simulink model "mod_sim_VTMS"  (R2018b)
settings: Solver=FixedStepDiscrete  StartTime=0.0  StopTime=t_Simulation  FixedStep=delta_t  RelTol=1e-3
values from neighbouring files (symbols this model uses):
  P_charge = 150    [main_sim_VTMS.m]
undefined symbols (not defined in the file or in its folder): A_EMaschine_Getriebe, A_j_c, A_Stirn, Anzahl_Peltierelemente, b_Batteriepack, b_c, b_EMaschine, b_Getriebe, b_j, b_Ladegeraet, BatPara, c_W, delta_t, DiscIntNeverNeededParam, e_Fahrzeug, eta_EMaschine_Break_M_EMaschine, eta_EMaschine_Break_n_EMaschine, eta_EMaschine_Faktor_Volllast, eta_EMaschine_Table, eta_Getriebe, eta_Ladegeraet, eta_Leistungselektronik_Break_M_EMaschine, eta_Leistungselektronik_Break_n_EMaschine, eta_Leistungselektronik_Faktor_Volllast, eta_Leistungselektronik_Table, f_R, I_DT_U_Break_DT, I_DT_U_Break_U, I_DT_U_Value_I, i_Getriebe, I_max, Ladevorgang, M_EMaschine_max, m_Fahrzeug, m_Zuladung, n_Zelle, P_Nebenverbraucher, p_Zelle, Peltier_Max_Eff, Q_DT_U_Break_DT, Q_DT_U_Break_U, Q_DT_U_Value_Q, Q_Imax_DT_Break_DT, Q_Imax_DT_Value_Q, r_dynamisch, rho_Luft, s_Zelle, SOC_init, Steuerung_Kuehlerluefter, Steuerung_Pumpe, Steuerung_Ventil, switch_BP_Zyklus, T_Batteriepack_init, T_EMaschine_Getriebe_init, T_Ladegeraet_init, T_Ladegeraet_Offset, T_Leistungselektronik_init, T_Offset_Batteriepack, T_Offset_EMaschine_Getriebe, T_Offset_Leistungselektronik ... (+36)
libraries: simulink x3, simulink_extras x2
(part 4 of 5)

== system mod_sim_VTMS/Thermomanagementsystem/Fluid/Fluid_Komponente thermisch/Konduktion 1. finites Volumen mit vorheriger Fluid_Komponente - Ventil ==
  note: PQ_FinitesVolumen_FinitesVolumen_1 = (T_FinitesVolumen_vor1_n - T_FinitesVolumen_1) / R_Ersatz
      | = Konduktion für das 1. finite Volumen mit vorherigem finiten Volumen
      |
      | mit R_Ersatz für Hauptpfad (Hauptpfad = 1) = R_FinitesVolumen / 2 + R_FinitesVolumen_vor1 / (2 * (1 - Zustand_Ventil)) = (R_FinitesVolumen + R_FinitesVolumen_vor1 / (1 - Zustand_Ventil)) / 2
      | mit R_Ersatz für Nebenpfad (Hauptpfad = 0) = R_FinitesVolumen / 2 + R_FinitesVolumen_vor1 / (2 * Zustand_Ventil) = (R_FinitesVolumen + R_FinitesVolumen_vor1 / Zustand_Ventil) / 2
      |
      | -> Dieses Subsystem repräsentiert den Fall, dass sich diese Fluid_Komponente sich nach einem Dreiwegeventil befindet
      | -> Diese Fluid_Komponente befindet sich nach 1 Fluid_Komponente + Fluid_Komponente vor dieser Fluid_Komponente befindet sich vor 2 Fluid_Komponenten
      | -> Diese Fluid_Komponente befindet sich entweder im Hauptpfad oder im Nebenpfad dieses Dreiwegeventils
      | -> Der Anwender legt in MATLAB fest, in welchem Pfad des Dreiwegeventils sich diese Fluid_Komponente befindet
      | -> Hauptpfad: Bei Zustand_Ventil = 0 fließt alles über den Hauptpfad, bei Zustand_Ventil = 1 fließt nichts über den Hauptpfad
      | -> Nebenpfad: Bei Zustand_Ventil = 0 fließt nichts über den Nebenpfad, bei Zustand_Ventil = 1 fließt alles über den Nebenpfad
      | -> Es gilt die Annahme: Diese Fluid_Komponente steht in Beziehung mit Zustand_Ventil (falls im Nebenpfad dieses Dreiwegeventils) bzw. mit (1 - Zustand_Ventil) (falls im Hauptpfad dieses Dreiwegeventils) der Querschnittsfläche der Kühlflüssigkeit in Fluid_Komponente_vor1
      |
      | -> Für die Herleitung dieses mathematischen Zusammenhangs wird auf die auf die im Rahmen des Thermomanagementsystemmodells erstellte Masterarbeit "Entwicklung und Steuerung eines Thermomanagementsystemmodells für Elektrofahrzeuge" verwiesen
  T_FinitesVolumen [K] : Inport
  R_FinitesVolumen [K*W^-1] : Inport  Port=2
  T_FinitesVolumen_vor1 [K] : Inport  Port=3
  R_FinitesVolumen_vor1 [K*W^-1] : Inport  Port=4
  Zustand_Ventil [-] : Inport  Port=5
  Add : Sum
  Constant : Constant  VectorParams1D=off
  Divide : Product  Inputs=*/
  Gain : Gain  Gain=0.5
  Hauptpfad : Constant  Value=0  VectorParams1D=off
  MATLAB Function : MATLAB Function  TreatAsAtomicUnit=on
  Subtract : Sum  Inputs=+-
  Switch : Switch  Criteria=u2 > Threshold
  PQ_FinitesVolumen_FinitesVolumen [W] : Outport
  wires:
  MATLAB Function/1(y) -> PQ_FinitesVolumen_FinitesVolumen [W]/1
  T_FinitesVolumen_vor1 [K]/1 -> MATLAB Function/2(v)
  R_FinitesVolumen_vor1 [K*W^-1]/1 -> Divide/1
  T_FinitesVolumen [K]/1 -> MATLAB Function/1(u)
  Divide/1 -> Add/2
  R_FinitesVolumen [K*W^-1]/1 -> Add/1
  Add/1 -> Gain/1
  Gain/1 -> MATLAB Function/3(a)
  Switch/1 -> Divide/2
  Zustand_Ventil [-]/1 -> Subtract/2, Switch/3
  Subtract/1 -> Switch/1
  Constant/1 -> Subtract/1
  Hauptpfad/1 -> Switch/2

== system mod_sim_VTMS/Thermomanagementsystem/Fluid/Fluid_Komponente thermisch/Konduktion 1. finites Volumen mit vorheriger Fluid_Komponente - normal ==
  note: PQ_FinitesVolumen_FinitesVolumen_1 = (T_FinitesVolumen_vor1_n - T_FinitesVolumen_1) / R_Ersatz
      | = Konduktion für das 1. finite Volumen mit vorherigem finiten Volumen
      |
      | mit R_Ersatz = R_FinitesVolumen / 2 + R_FinitesVolumen_vor1 / 2 = (R_FinitesVolumen + R_FinitesVolumen_vor1) / 2
      |
      | -> Dieses Subsystem repräsentiert den Fall, dass sich diese Fluid_Komponente nach einer anderen Fluid_Komponente ohne Dreiwegeventil oder Vereinigung der zwei nach der Aufzweigung durch ein Dreiwegeventil resultierenden Pfade befindet
      | -> Diese Fluid_Komponente befindet sich nach 1 Fluid_Komponente + Fluid_Komponente vor dieser Fluid_Komponente befindet sich vor 1 Fluid_Komponente
      |
      | -> Für die Herleitung dieses mathematischen Zusammenhangs wird auf die auf die im Rahmen des Thermomanagementsystemmodells erstellte Masterarbeit "Entwicklung und Steuerung eines Thermomanagementsystemmodells für Elektrofahrzeuge" verwiesen
  T_FinitesVolumen [K] : Inport
  R_FinitesVolumen [K*W^-1] : Inport  Port=2
  T_FinitesVolumen_vor1 [K] : Inport  Port=3
  R_FinitesVolumen_vor1 [K*W^-1] : Inport  Port=4
  Add : Sum
  Gain : Gain  Gain=0.5
  MATLAB Function : MATLAB Function  TreatAsAtomicUnit=on
  PQ_FinitesVolumen_FinitesVolumen [W] : Outport
  wires:
  R_FinitesVolumen_vor1 [K*W^-1]/1 -> Add/2
  T_FinitesVolumen_vor1 [K]/1 -> MATLAB Function/2(v)
  MATLAB Function/1(y) -> PQ_FinitesVolumen_FinitesVolumen [W]/1
  R_FinitesVolumen [K*W^-1]/1 -> Add/1
  Add/1 -> Gain/1
  T_FinitesVolumen [K]/1 -> MATLAB Function/1(u)
  Gain/1 -> MATLAB Function/3(a)

== system mod_sim_VTMS/Thermomanagementsystem/Fluid/Fluid_Komponente thermisch/Konduktion finite Volumen innerhalb Fluid_Komponente ==
  note: PQ_FinitesVolumen_FinitesVolumen_i = (T_FinitesVolumen_i-1 - T_FinitesVolumen_i) / R_FinitesVolumen + (T_FinitesVolumen_i+1 - T_FinitesVolumen_i) / R_FinitesVolumen für i = 2 ... n-1
      | = (T_FinitesVolumen_i-1 + T_FinitesVolumen_i+1 - 2 * T_FinitesVolumen_i) / R_FinitesVolumen für i = 2 ... n-1
      | = Konduktion für das i. finite Volumen mit vorherigem und nachfolgendem finiten Volumen für i = 2 ... n-1
      |
      | PQ_FinitesVolumen_FinitesVolumen_1 = (T_FinitesVolumen_2 - T_FinitesVolumen_1) / R_FinitesVolumen
      | = Konduktion für das 1. finite Volumen mit nachfolgendem finiten Volumen
      |
      | PQ_FinitesVolumen_FinitesVolumen_n = (T_FinitesVolumen_n-1 - T_FinitesVolumen_n) / R_FinitesVolumen
      | = Konduktion für das n. finite Volumen mit vorherigem finiten Volumen
      |
      | -> Der Widerstand zwischen den einzelnen Knoten der finiten Volumen ist jeweils R_FinitesVolumen, weil die Wärmeleitfähigkeit und die Querschnittsfläche der Kühlflüssigkeit innerhalb einer Fluid_Komponente identisch sind und der Abstand zwischen den einzelnen Knoten gleich der Länge eines finiten Volumen ist
      | -> Die Bestimmung der Konduktion für ein finites Volumen mit vorherigem und nachfolgenden finiten Volumen ist innerhalb einer Fluid_Komponente nur für i = 2 ... n-1 möglich, weil das 1. bzw. n. finite Volumen einer Fluid_Komponente nur Konduktion mit dem 2. (nachfolgenden) bzw. n-1. (vorherigem) finten Volumen derselben Fluid_Komponente hat
      | -> Die restliche Konduktion für das 1. und n. finite Volumen finden mit anderen Fluid_Komponenten statt und werden deswegen durch die Kopplungsfälle dargestellt
      |
      | -> Für die Herleitung dieser mathematischen Zusammenhänge wird auf die auf die im Rahmen des Thermomanagementsystemmodells erstellte Masterarbeit "Entwicklung und Steuerung eines Thermomanagementsystemmodells für Elektrofahrzeuge" verwiesen
      |
      | -> Für die Herleitung dieses mathematischen Zusammenhangs wird auf die auf die im Rahmen des Thermomanagementsystemmodells erstellte Masterarbeit "Entwicklung und Steuerung eines Thermomanagementsystemmodells für Elektrofahrzeuge" verwiesen
      | -> Für die Herleitung dieses mathematischen Zusammenhangs wird auf die auf die im Rahmen des Thermomanagementsystemmodells erstellte Masterarbeit "Entwicklung und Steuerung eines Thermomanagementsystemmodells für Elektrofahrzeuge" verwiesen
      | -> Für die Herleitung dieses mathematischen Zusammenhangs wird auf die auf die im Rahmen des Thermomanagementsystemmodells erstellte Masterarbeit "Entwicklung und Steuerung eines Thermomanagementsystemmodells für Elektrofahrzeuge" verwiesen
  T_FinitesVolumen [K] : Inport
  R_FinitesVolumen [K*W^-1] : Inport  Port=2
  MATLAB Function : MATLAB Function  TreatAsAtomicUnit=on
  PQ_FinitesVolumen_FinitesVolumen [W] : Outport
  wires:
  T_FinitesVolumen [K]/1 -> MATLAB Function/1(u)
  R_FinitesVolumen [K*W^-1]/1 -> MATLAB Function/2(a)
  MATLAB Function/1(y) -> PQ_FinitesVolumen_FinitesVolumen [W]/1

== system mod_sim_VTMS/Thermomanagementsystem/Fluid/Fluid_Komponente thermisch/Konduktion n. finites Volumen mit nachfolgenden Fluid_Komponenten - Ventil ==
  note: PQ_FinitesVolumen_FinitesVolumen_n = (T_FinitesVolumen_nach1_1 - T_FinitesVolumen_n) / R_Ersatz_1 + (T_FinitesVolumen_nach2_1 - T_FinitesVolumen_n) / R_Ersatz_2
      | = Konduktion für das n. finite Volumen mit nachfolgendem finiten Volumen
      |
      | mit R_Ersatz_1 = R_FinitesVolumen / (2 * (1 - Zustand_Ventil)) + R_FinitesVolumen_nach1 / 2 = (R_FinitesVolumen / (1 - Zustand_Ventil) + R_FinitesVolumen_nach1) / 2 -> Fluid_Komponente_nach1 befindet sich im Hauptpfad des Dreiwegeventils
      | mit R_Ersatz_2 = R_FinitesVolumen / (2 * Zustand_Ventil) + R_FinitesVolumen_nach1 / 2 = (R_FinitesVolumen / Zustand_Ventil + R_FinitesVolumen_nach2) / 2 -> Fluid_Komponente_nach2 befindet sich im Nebenpfad des Dreiwegeventils
      |
      | -> Dieses Subsystem repräsentiert den Fall, dass sich diese Fluid_Komponente vor einem Dreiwegeventil befindet
      | -> Diese Fluid_Komponente befindet sich vor 2 Fluid_Komponenten
      | -> Eine der nachfolgenden Fluid_Komponenten befindet sich im Hauptpfad dieses Dreiwegeventils und die andere nachfolgende Fluid_Komponente im Nebenpfad dieses Dreiwegeventil
      | -> Der Anwender legt in MATLAB fest, in welchem Pfad des Dreiwegeventils sich die nachfolgenden Fluid_Komponenten befinden
      | -> Fluid_Komponente_nach1 befindet sich im Hauptpfad dieses Dreiwegeventils, Fluid_Komponente_nach2 befindet sich im Nebenpfad dieses Dreiwegeventils
      | -> Hauptpfad: Bei Zustand_Ventil = 0 fließt alles über den Hauptpfad, bei Zustand_Ventil = 1 fließt nichts über den Hauptpfad
      | -> Nebenpfad: Bei Zustand_Ventil = 0 fließt nichts über den Nebenpfad, bei Zustand_Ventil = 1 fließt alles über den Nebenpfad
      | -> Es gilt die Annahme: Diese Fluid_Komponente steht mit (1 - Zustand_Ventil) ihrer Querschnittsfläche der Kühlflüssigkeit in Beziehung mit Fluid_Komponente_nach1 und mit Zustand_Ventil ihrer Querschnittsfläche der Kühlflüssigkeit in Beziehnung mit Fluid_Komponente_nach2
      |
      | -> Für die Herleitung dieses mathematischen Zusammenhangs wird auf die auf die im Rahmen des Thermomanagementsystemmodells erstellte Masterarbeit "Entwicklung und Steuerung eines Thermomanagementsystemmodells für Elektrofahrzeuge" verwiesen
  T_FinitesVolumen [K] : Inport
  R_FinitesVolumen [K*W^-1] : Inport  Port=2
  T_FinitesVolumen_nach1 [K] : Inport  Port=3
  R_FinitesVolumen_nach1 [K*W^-1] : Inport  Port=4
  T_FinitesVolumen_nach2 [K] : Inport  Port=5
  R_FinitesVolumen_nach2 [K*W^-1] : Inport  Port=6
  Zustand_Ventil [-] : Inport  Port=7
  Add : Sum
  Add1 : Sum
  Constant : Constant
  Divide : Product  Inputs=*/
  Divide1 : Product  Inputs=*/
  Gain : Gain  Gain=0.5
  Gain1 : Gain  Gain=0.5
  MATLAB Function : MATLAB Function  TreatAsAtomicUnit=on
  Subtract : Sum  Inputs=+-
  PQ_FinitesVolumen_FinitesVolumen [W] : Outport
  wires:
  R_FinitesVolumen [K*W^-1]/1 -> Divide1/1, Divide/1
  Add/1 -> Gain/1
  Divide/1 -> Add/1
  MATLAB Function/1(y) -> PQ_FinitesVolumen_FinitesVolumen [W]/1
  T_FinitesVolumen [K]/1 -> MATLAB Function/1(u)
  T_FinitesVolumen_nach2 [K]/1 -> MATLAB Function/3(w)
  T_FinitesVolumen_nach1 [K]/1 -> MATLAB Function/2(v)
  Gain/1 -> MATLAB Function/4(a)
  Subtract/1 -> Divide/2
  Constant/1 -> Subtract/1
  R_FinitesVolumen_nach1 [K*W^-1]/1 -> Add/2
  Add1/1 -> Gain1/1
  Divide1/1 -> Add1/1
  Gain1/1 -> MATLAB Function/5(b)
  R_FinitesVolumen_nach2 [K*W^-1]/1 -> Add1/2
  Zustand_Ventil [-]/1 -> Divide1/2, Subtract/2

== system mod_sim_VTMS/Thermomanagementsystem/Fluid/Fluid_Komponente thermisch/Konduktion n. finites Volumen mit nachfolgender Fluid_Komponente - Vereinigung ==
  note: PQ_FinitesVolumen_FinitesVolumen_n = (T_FinitesVolumen_nach1_1 - T_FinitesVolumen_n) / R_Ersatz
      | = Konduktion für das n. finite Volumen mit nachfolgendem finiten Volumen
      |
      | mit R_Ersatz = R_FinitesVolumen / 2 + R_FinitesVolumen_nach1 / (2 * 0.5) = R_FinitesVolumen / 2 + R_FinitesVolumen_nach1
      |
      | -> Dieses Subsystem repäsentiert den Fall, dass sich diese Fluid_Komponente vor der Vereinigung der zwei nach der Aufzweigung durch ein Dreiwegeventil resultierenden Pfade befindet
      | -> Diese Fluid_Komponente befindet sich vor 1 Fluid_Komponente + Fluid_Komponente nach dieser Fluid_Komponente befindet sich nach 2 Fluid_Komponenten
      | -> Diese Fluid_Komponente befindet sich in einem der Pfade dieses Dreiwegeventils (es ist egal, in welchem Pfad dieses Dreiwegeventils, weil das Prinzip der Berechnung gleich ist -> siehe unten)
      | -> Nach dieser Fluid_Komponente befindet sich kein Dreiwegeventil mit einem bestimmten Zustand, sondern es gilt die Annahme: Diese Fluid_Komponente steht in Beziehung mit 50% der Querschnittsfläche der Kühlflüssigkeit in Fluid_Komponente_nach1
      |
      | -> Für die Herleitung dieses mathematischen Zusammenhangs wird auf die auf die im Rahmen des Thermomanagementsystemmodells erstellte Masterarbeit "Entwicklung und Steuerung eines Thermomanagementsystemmodells für Elektrofahrzeuge" verwiesen
  T_FinitesVolumen [K] : Inport
  R_FinitesVolumen [K*W^-1] : Inport  Port=2
  T_FinitesVolumen_nach1 [K] : Inport  Port=3
  R_FinitesVolumen_nach1 [K*W^-1] : Inport  Port=4
  Add1 : Sum
  Gain1 : Gain  Gain=0.5
  MATLAB Function : MATLAB Function  TreatAsAtomicUnit=on
  PQ_FinitesVolumen_FinitesVolumen [W] : Outport
  wires:
  T_FinitesVolumen_nach1 [K]/1 -> MATLAB Function/2(v)
  MATLAB Function/1(y) -> PQ_FinitesVolumen_FinitesVolumen [W]/1
  T_FinitesVolumen [K]/1 -> MATLAB Function/1(u)
  R_FinitesVolumen_nach1 [K*W^-1]/1 -> Add1/2
  R_FinitesVolumen [K*W^-1]/1 -> Gain1/1
  Gain1/1 -> Add1/1
  Add1/1 -> MATLAB Function/3(a)

== system mod_sim_VTMS/Thermomanagementsystem/Fluid/Fluid_Komponente thermisch/Konduktion n. finites Volumen mit nachfolgender Fluid_Komponente - normal ==
  note: PQ_FinitesVolumen_FinitesVolumen_n = (T_FinitesVolumen_nach1_1 - T_FinitesVolumen_n) / R_Ersatz
      | = Konduktion für das n. finite Volumen mit nachfolgendem finiten Volumen
      |
      | mit R_Ersatz = R_FinitesVolumen / 2 + R_FinitesVolumen_nach1 / 2 = (R_FinitesVolumen + R_FinitesVolumen_nach1) / 2
      |
      | -> Dieses Subsystem repräsentiert den Fall, dass sich diese Fluid_Komponente vor einer anderen Fluid_Komponente ohne Dreiwegeventil oder Vereinigung der zwei nach der Aufzweigung durch ein Dreiwegeventil resultierenden Pfade befindet
      | -> Diese Fluid_Komponente befindet sich vor 1 Fluid_Kompnente + Fluid_Komponente nach dieser Fluid_Komponente befindet sich nach 1 Fluid_Komponente
      |
      | -> Für die Herleitung dieses mathematischen Zusammenhangs wird auf die auf die im Rahmen des Thermomanagementsystemmodells erstellte Masterarbeit "Entwicklung und Steuerung eines Thermomanagementsystemmodells für Elektrofahrzeuge" verwiesen
  T_FinitesVolumen [K] : Inport
  R_FinitesVolumen [K*W^-1] : Inport  Port=2
  T_FinitesVolumen_nach1 [K] : Inport  Port=3
  R_FinitesVolumen_nach1 [K*W^-1] : Inport  Port=4
  Add : Sum
  Gain : Gain  Gain=0.5
  MATLAB Function : MATLAB Function  TreatAsAtomicUnit=on
  PQ_FinitesVolumen_FinitesVolumen [W] : Outport
  wires:
  MATLAB Function/1(y) -> PQ_FinitesVolumen_FinitesVolumen [W]/1
  Gain/1 -> MATLAB Function/3(a)
  T_FinitesVolumen [K]/1 -> MATLAB Function/1(u)
  R_FinitesVolumen_nach1 [K*W^-1]/1 -> Add/2
  R_FinitesVolumen [K*W^-1]/1 -> Add/1
  T_FinitesVolumen_nach1 [K]/1 -> MATLAB Function/2(v)
  Add/1 -> Gain/1

== system mod_sim_VTMS/Thermomanagementsystem/Kühler/Kuehler thermisch/Bestimmung v_Kuehlerluefter ==
  note: -> Ein Kühlerlüfter wird nicht modelliert
      | -> Es wird nur die Luftgeschwindigkeit eines Kühlerlüfters benötigt
      | -> Kühlerlüfter gesteuert (Steuerung_Kuehlerluefter = 1): v_Kuehlerluefter wird über Steuerung in Subsystem "Steuerung Kuehlerluefter" bestimmt
      | -> Kühlerlüfter ungesteuert (Steuerung_Kuehlerluefter = 0): v_Kuehlerluefter wird zeitabhängig vom Anwender vorgegeben
  note: -> Ein Kühler besitzt einen Kühlerlüfter, der den Kühler mit seiner Luftgeschwindigkeit anströmt
      | -> Ein Kühlerlüfter wird als 0D angenommen
      | -> Je nachdem wie es der Anwender wünscht, können Kühlerlüfter gesteuert oder ungesteuert sein
  T_FinitesVolumen [K] : Inport
  Constant : Constant  Value=Steuerung_Kuehlerluefter  VectorParams1D=off
  Steuerung Kuehlerluefter : Subsystem
  Switch : Switch  Criteria=u2 > Threshold
  v_Kuehlerluefter : FromWorkspace  VariableName=[0,0]  SampleTime=0
  v_Kuehlerluefter [m*s^-1] : Outport
  wires:
  Switch/1 -> v_Kuehlerluefter [m*s^-1]/1
  Constant/1 -> Switch/2
  v_Kuehlerluefter/1 -> Switch/3
  Steuerung Kuehlerluefter/1(v_Kuehlerluefter [m*s^-1]) -> Switch/1
  T_FinitesVolumen [K]/1 -> Steuerung Kuehlerluefter/1(T_FinitesVolumen [K])

== system mod_sim_VTMS/Thermomanagementsystem/Ladegeraet/Ladegeraet(1) elektrisch/Fast charging control ==
  note: Current reduction step in W
      | if max voltage is reached
  U_cell [V] : Inport
  Enable : EnablePort  StatesWhenEnabling=reset
  Add1 : Sum  Inputs=+-
  Charging Power : UnitDelay  InitialCondition=P_charge*1000  SampleTime=-1
  Constant2 : Constant  Value=100
  Constant3 : Constant  Value=0
  Saturation : Saturate  UpperLimit=inf  LowerLimit=0
  Switch1 : Switch  Threshold=4.18
  charging power [W] : Outport  OutputWhenDisabled=reset  InitialOutput=0
  wires:
  Constant2/1 -> Switch1/1
  Constant3/1 -> Switch1/3
  Add1/1 -> Saturation/1
  Switch1/1 -> Add1/2
  U_cell [V]/1 -> Switch1/2
  Charging Power/1 -> Add1/1
  Saturation/1 -> charging power [W]/1, Charging Power/1

== system mod_sim_VTMS/Thermomanagementsystem/Ladegeraet/Ladegeraet(1) thermisch/Waermeaustausch Ladegeraet - Fluid ==
  note: PQ_Ladegeraet_FinitesVolumen_i = UA_Ladegeraet_FinitesVolumen * (T_Ladegeraet - T_FinitesVolumen_i) für i = 1:n
      | PQ_Ladegeraet_Kuehlfluessigkeit = Summe (PQ_Ladegeraet_FinitesVolumen_i) für i = 1:n
      |
      | mit UA_Ladegeraet_FinitesVolumen = f (PV_Kuehlfluessigkeit)
      |
      | -> UA_Ladegeraet_FinitesVolumen und T_Ladegeraet ist für jedes finite Volumen des Fluids im Ladegeraet identisch, weil das Ladegeraet als Punktmasse betrachtet wird
      |
      | -> Deswegen ergibt sich die Wärmeleistung bzgl. dem Ladegeraet über den Wärmeaustausch mit der gesamten Kühlflüssigkeit, was der Summe aus den Wärmeaustauschen mit den finiten Volumen entspricht
  T_Ladegeraet [K] : Inport
  T_FinitesVolumen [K] : Inport  Port=2
  PV_Ladegeraet [m^3*s^-1] : Inport  Port=3
  1-D Lookup Table : Lookup_n-D  NumberOfTableDimensions=1  BreakpointsForDimension1=UA_Ladegeraet_FinitesVolumen_Break_PV_Kuehlfluessigkeit{1}  BeginIndexSearchUsingPreviousIndexResult=on  Table=UA_Ladegeraet_FinitesVolumen_Table{1}  ExtrapMethod=Clip  UseLastTableValue=on  InternalRulePriority=Speed  RndMeth=Simplest  InputSameDT=on
  Matrix Sum : Sum  Inputs=+
  Product : Product
  Subtract : Sum  Inputs=+-
  PQ_Ladegeraet_Kuehlfluessigkeit [W] : Outport
  PQ_Ladegeraet_FinitesVolumen [W] : Outport  Port=2
  wires:
  1-D Lookup Table/1 -> Product/1  "UA_Ladegeraet_FinitesVolumen [W*K^-1]"
  T_Ladegeraet [K]/1 -> Subtract/1
  Subtract/1 -> Product/2
  Matrix Sum/1 -> PQ_Ladegeraet_Kuehlfluessigkeit [W]/1
  Product/1 -> PQ_Ladegeraet_FinitesVolumen [W]/1, Matrix Sum/1
  PV_Ladegeraet [m^3*s^-1]/1 -> 1-D Lookup Table/1
  T_FinitesVolumen [K]/1 -> Subtract/2

== system mod_sim_VTMS/Thermomanagementsystem/Ladegeraet/Ladegeraet(1) thermisch/Waermeaustausch Ladegeraet - Umgebung  ==
  note: PQ_Ladegeraet_Umgebung = UA_Ladegeraet_Umgebung * (T_Ladegeraet - T_Umgebung_Offset)
      |
      | mit UA_Ladegeraet_Umgebung = f (v_Fahrzeug)
      | mit T_Umgebung_Offset = T_Umgebung + T_Ladegeraet_Offset
      |
      | -> Da die Umgebungstemperatur konstant ist, wird über T_Ladegeraet_Offset die Umgebungstemperatur um das Batteriepack manuell erhöht
  T_Ladegeraet [K] : Inport
  T_Umgebung_Offset [K] : Inport  Port=2
  v_Fahrzeug [m*s^-1] : Inport  Port=3
  1-D Lookup Table : Lookup_n-D  NumberOfTableDimensions=1  BreakpointsForDimension1=UA_Ladegeraet_Umgebung_Break_v_Fahrzeug{1}  BeginIndexSearchUsingPreviousIndexResult=on  Table=UA_Ladegeraet_Umgebung_Table{1}  ExtrapMethod=Clip  UseLastTableValue=on  InternalRulePriority=Speed  RndMeth=Simplest  InputSameDT=on
  Product1 : Product
  Subtract : Sum  Inputs=+-
  PQ_Ladegeraet_Umgebung [W] : Outport
  wires:
  T_Ladegeraet [K]/1 -> Subtract/1
  T_Umgebung_Offset [K]/1 -> Subtract/2
  Product1/1 -> PQ_Ladegeraet_Umgebung [W]/1
  1-D Lookup Table/1 -> Product1/1  "UA_Ladegeraet_Umgebung [W*K^-1]"
  Subtract/1 -> Product1/2
  v_Fahrzeug [m*s^-1]/1 -> 1-D Lookup Table/1

== system mod_sim_VTMS/Thermomanagementsystem/Leistungselektronik/Leistungselektronik(1) thermisch/Waermeaustausch Case - Kuehlfluessigkeit ==
  note: PQ_c_FinitesVolumen_i = UA_c_FinitesVolumen * (T_c - T_FinitesVolumen_i) für i = 1:n
      | PQ_c_Kuehlfluessigkeit = Summe (PQ_c_FinitesVolumen_i) für i = 1:n
      |
      | mit UA_c_FinitesVolumen = f (PV_Kuehlfluessigkeit)
      |
      | -> UA_c_FinitesVolumen ist für jedes finite Volumen des Strömungsgebiets der Leistungselektronik identisch, weil das Strömungsgebiet der Leistungselektronik durch identische finite Volumen örtlich diskretisiert ist und weil im gesamten Strömungsgebiet der Leistungselektronik der gleiche Volumenstrom der Kühlflüssigkeit vorliegt
      | -> T_c ist für jedes finite Volumen des Strömungsgebiets der Leistungselektronik identisch, weil die Case der MOSFET als Blockkapazität aufgefasst werden
      | -> Der Wärmestrom zwischen der/den Leistungselektronik/Case der MOSFET und der gesamten Kühlflüssigkeit im Strömungsgebiet der Leistungselektronik (wird für die thermische Modellierung der Leistungselektronik/Case der MOSFET benötigt) ergibt sich über die Summe aus den einzelnen Wärmeströmen zwischen d er/den Leistungselektronik/Case der MOSFET und der Kühlflüssigkeit in einem finiten Volumen des Strömungsgebiets der Leistungselektronik
  T_c [K] : Inport
  T_FinitesVolumen [K] : Inport  Port=2
  PV_Kuehlfluessigkeit [m^3*s^-1] : Inport  Port=3
  1-D Lookup Table : Lookup_n-D  NumberOfTableDimensions=1  BreakpointsForDimension1=UA_c_FinitesVolumen_Break_PV_Kuehlfluessigkeit{1}  BeginIndexSearchUsingPreviousIndexResult=on  Table=UA_c_FinitesVolumen_Table{1}  ExtrapMethod=Clip  UseLastTableValue=on  InternalRulePriority=Speed  RndMeth=Simplest  InputSameDT=on
  Matrix Sum : Sum  Inputs=+
  Product : Product
  Subtract : Sum  Inputs=+-
  PQ_c_Kuehlfluessigkeit [W] : Outport
  PQ_c_FinitesVolumen [W] : Outport  Port=2
  wires:
  Product/1 -> PQ_c_FinitesVolumen [W]/1, Matrix Sum/1
  Subtract/1 -> Product/2
  T_c [K]/1 -> Subtract/1
  Matrix Sum/1 -> PQ_c_Kuehlfluessigkeit [W]/1
  PV_Kuehlfluessigkeit [m^3*s^-1]/1 -> 1-D Lookup Table/1
  1-D Lookup Table/1 -> Product/1  "UA_c_FinitesVolumen [W*K^-1]"
  T_FinitesVolumen [K]/1 -> Subtract/2

== system mod_sim_VTMS/Thermomanagementsystem/Leistungselektronik/Leistungselektronik(1) thermisch/Waermeaustausch Case - Umgebungsluft ==
  note: PQ_c_Umgebung = UA_c_Umgebung * (T_c - T_Umgebung_Leistungselektronik)
      |
      | mit UA_c_Umgebung = f (v_Fahrzeug)
      | mit T_Umgebung_Leistungselektronik = T_Umgebung + T_Offset_Leistungselektronik
      |
      | -> Durch T_Offset_Leistungselektronik ist die Temperatur der Umgebungsluft um die Leistungselektronik/Case der MOSFET zur normalen Temperatur der Umgebungsluft verändert
  T_c [K] : Inport
  T_Umgebung_Leistungselektronik [K] : Inport  Port=2
  v_Fahrzeug [m*s^-1] : Inport  Port=3
  1-D Lookup Table : Lookup_n-D  NumberOfTableDimensions=1  BreakpointsForDimension1=UA_c_Umgebung_Break_v_Fahrzeug{1}  BeginIndexSearchUsingPreviousIndexResult=on  Table=UA_c_Umgebung_Table{1}  ExtrapMethod=Clip  UseLastTableValue=on  InternalRulePriority=Speed  RndMeth=Simplest  InputSameDT=on
  Product : Product
  Subtract : Sum  Inputs=+-
  PQ_c_Umgebung [W] : Outport
  wires:
  T_c [K]/1 -> Subtract/1
  1-D Lookup Table/1 -> Product/1  "UA_c_Umgebung [W*K^-1]"
  Subtract/1 -> Product/2
  Product/1 -> PQ_c_Umgebung [W]/1
  T_Umgebung_Leistungselektronik [K]/1 -> Subtract/2
  v_Fahrzeug [m*s^-1]/1 -> 1-D Lookup Table/1

== system mod_sim_VTMS/Thermomanagementsystem/PCM/PCM thermisch/Phasenuebergang ==
  note: In diesem Block wird abgeglichen, ob sich die Temperatur der Komponente im Bereich des Phasenübergangs befindet.
      | Da für den Phasenwechsel Energie in Form der Schmelz- und Erstarrungsenthalpie benötigt wird, steigt die Temperatur langsamer an, dies wird durch den Faktor_PW dargestellt.
      | Handelt es sich bei diesem um ein aktivierbares PCM, einen Latenwärmespeicher, findet der Phasenwechsel bereits komplett bei dessen Aktivierung statt. Deswegen kühlt das PCM im aktivierten Zustand mit normaler Rate ab, obwohl sie sich im Temperaturbereich des Phasenübergangs befindet. Der Zustand wird über das Signal PW_ausgesetzt übermittelt und unterbricht im aktivierten Fall das Steuerungsignal für die reduzierte Temperaturdifferenz im Bereich des Phasenübergangs.
  Temp : Inport
  dT_in : Inport  Port=2
  Trigger_aktiv : Inport  Port=3
  Faktor_Phasenwechsel : Constant  Value=0.1  VectorParams1D=off
  Logical Operator1 : Logic  AllPortsSameDT=off  OutDataTypeStr=boolean
  Logical Operator2 : Logic  AllPortsSameDT=off  OutDataTypeStr=boolean
  Logical Operator3 : Logic  Operator=NOT  AllPortsSameDT=off  OutDataTypeStr=boolean
  Phasenwechsel_oGW : Constant  Value=333.15  VectorParams1D=off
  Phasenwechsel_uGW : Constant  Value=331.15  VectorParams1D=off
  Product : Product
  Relational Operator1 : RelationalOperator  Operator=<  OutDataTypeStr=boolean  RndMeth=Simplest
  Relational Operator2 : RelationalOperator  Operator=<=  OutDataTypeStr=boolean  RndMeth=Simplest
  Switch6 : Switch  Criteria=u2 ~= 0  Threshold=56
  dT_out : Outport
  wires:
  Temp/1 -> Relational Operator2/1, Relational Operator1/2
  Relational Operator2/1 -> Logical Operator1/2
  Relational Operator1/1 -> Logical Operator1/1
  dT_in/1 -> Product/2, Switch6/3
  Phasenwechsel_uGW/1 -> Relational Operator1/1
  Switch6/1 -> dT_out/1
  Phasenwechsel_oGW/1 -> Relational Operator2/2
  Product/1 -> Switch6/1
  Faktor_Phasenwechsel/1 -> Product/1
  Trigger_aktiv/1 -> Logical Operator3/1
  Logical Operator1/1 -> Logical Operator2/1
  Logical Operator2/1 -> Switch6/2
  Logical Operator3/1 -> Logical Operator2/2

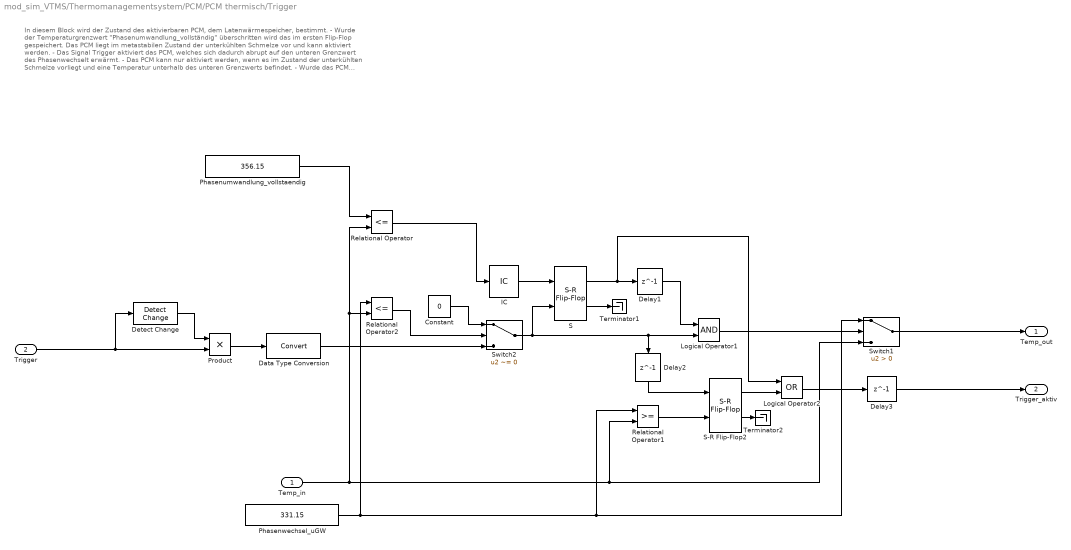
== system mod_sim_VTMS/Thermomanagementsystem/PCM/PCM thermisch/Trigger ==
  note: In diesem Block wird der Zustand des aktivierbaren PCM, dem Latenwärmespeicher, bestimmt.
      | - Wurde der Temperaturgrenzwert "Phasenumwandlung_vollständig" überschritten wird das im ersten Flip-Flop gespeichert. Das PCM liegt im metastabilen Zustand der unterkühlten Schmelze vor und kann aktiviert werden.
      | - Das Signal Trigger aktiviert das PCM, welches sich dadurch abrupt auf den unteren Grenzwert des Phasenwechselt erwärmt.
      | - Das PCM kann nur aktiviert werden, wenn es im Zustand der unterkühlten Schmelze vorliegt und eine Temperatur unterhalb des unteren Grenzwerts befindet.
      | - Wurde das PCM aktiviert wird ein Signal "PW_ausgesetzt" an den Block Phasenübergang weitergegeben, um wiederzugeben, dass der Phasenübergang bereits passiert ist und keine verlangsamte Abkühlung stattfindet. Dieses Signal stellt sich wieder auf null, wenn sich die Temperatur des PCM wieder unterhalb des unteren Grenzwerts befindet.
  Temp_in : Inport
  Trigger : Inport  Port=2
  Constant : Constant  Value=0  OutDataTypeStr=boolean
  Data Type Conversion : DataTypeConversion
  Delay1 : Delay  DelayLength=1  InitialCondition=1
  Delay2 : Delay  DelayLength=1  InitialCondition=0
  Delay3 : Delay  DelayLength=1  InitialCondition=0
  Detect Change : simulink/Logic and Bit Operations/Detect Change  vinit=0  OutDataTypeStr=boolean
  IC : InitialCondition
  Logical Operator1 : Logic  AllPortsSameDT=off  OutDataTypeStr=boolean
  Logical Operator2 : Logic  Operator=OR  AllPortsSameDT=off  OutDataTypeStr=boolean
  Phasenumwandlung_vollstaendig : Constant  Value=356.15  VectorParams1D=off
  Phasenwechsel_uGW : Constant  Value=331.15  VectorParams1D=off
  Product : Product
  Relational Operator : RelationalOperator  Operator=<=  OutDataTypeStr=boolean  RndMeth=Simplest
  Relational Operator1 : RelationalOperator  OutDataTypeStr=boolean  RndMeth=Simplest
  Relational Operator2 : RelationalOperator  Operator=<=  OutDataTypeStr=boolean  RndMeth=Simplest
  S : simulink_extras/Flip Flops/S-R Flip-Flop  initial_condition=0
  S-R Flip-Flop2 : simulink_extras/Flip Flops/S-R Flip-Flop  initial_condition=0
  Switch1 : Switch  Criteria=u2 > Threshold
  Switch2 : Switch  Criteria=u2 ~= 0
  Terminator1 : Terminator
  Terminator2 : Terminator
  Temp_out : Outport
  Trigger_aktiv : Outport  Port=2
  wires:
  Temp_in/1 -> Relational Operator1/2, Switch1/3, Relational Operator/2, Relational Operator2/2
  Switch2/1 -> Delay2/1, Logical Operator1/2, S/2
  Switch1/1 -> Temp_out/1
  Phasenumwandlung_vollstaendig/1 -> Relational Operator/1
  S/2 -> Terminator1/1
  S/1 -> Logical Operator2/1, Delay1/1
  Logical Operator1/1 -> Switch1/2
  Trigger/1 -> Product/2, Detect Change/1
  Detect Change/1 -> Product/1
  Product/1 -> Data Type Conversion/1
  Constant/1 -> Switch2/1
  Data Type Conversion/1 -> Switch2/3
  S-R Flip-Flop2/2 -> Terminator2/1
  Delay2/1 -> S-R Flip-Flop2/1
  Phasenwechsel_uGW/1 -> Relational Operator1/1, Switch1/1, Relational Operator2/1
  Relational Operator1/1 -> S-R Flip-Flop2/2
  IC/1 -> S/1
  Relational Operator/1 -> IC/1
  Delay3/1 -> Trigger_aktiv/1
  Relational Operator2/1 -> Switch2/2
  S-R Flip-Flop2/1 -> Logical Operator2/2
  Logical Operator2/1 -> Delay3/1
  Delay1/1 -> Logical Operator1/1

== system mod_sim_VTMS/Thermomanagementsystem/PCM/PCM thermisch/Waermeaustausch PCM - Fluid ==
  note: PQ_PCM_FinitesVolumen_i = UA_PCM_FinitesVolumen * (T_PCM - T_FinitesVolumen_i) für i = 1:n
      | PQ_PCM_Kuehlfluessigkeit = Summe (PQ_PCM_FinitesVolumen_i) für i = 1:n
      |
      | mit UA_PCM_FinitesVolumen = f (PV_Kuehlfluessigkeit)
      |
      | -> UA_PCM_FinitesVolumen und T_PCM ist für jedes finite Volumen des Fluids im PCM identisch, weil das PCM als Punktmasse betrachtet wird
      |
      | -> Deswegen ergibt sich die Wärmeleistung bzgl. dem PCM über den Wärmeaustausch mit der gesamten Kühlflüssigkeit, was der Summe aus den Wärmeaustauschen mit den finiten Volumen entspricht
  T_PCM [K] : Inport
  T_FinitesVolumen [K] : Inport  Port=2
  PV_PCM [m^3*s^-1] : Inport  Port=3
  1-D Lookup Table : Lookup_n-D  NumberOfTableDimensions=1  BreakpointsForDimension1=UA_PCM_FinitesVolumen_Break_PV_Kuehlfluessigkeit{1}  BeginIndexSearchUsingPreviousIndexResult=on  Table=UA_PCM_FinitesVolumen_Table{1}  ExtrapMethod=Clip  UseLastTableValue=on  InternalRulePriority=Speed  RndMeth=Simplest  InputSameDT=on
  Matrix Sum : Sum  Inputs=+
  Product : Product
  Subtract : Sum  Inputs=+-
  PQ_PCM_Kuehlfluessigkeit [W] : Outport
  PQ_PCM_FinitesVolumen [W] : Outport  Port=2
  wires:
  T_FinitesVolumen [K]/1 -> Subtract/2
  PV_PCM [m^3*s^-1]/1 -> 1-D Lookup Table/1
  Product/1 -> Matrix Sum/1, PQ_PCM_FinitesVolumen [W]/1
  Matrix Sum/1 -> PQ_PCM_Kuehlfluessigkeit [W]/1
  Subtract/1 -> Product/2
  T_PCM [K]/1 -> Subtract/1
  1-D Lookup Table/1 -> Product/1  "UA_PCM_FinitesVolumen [W*K^-1]"

== system mod_sim_VTMS/Thermomanagementsystem/PCM/PCM thermisch/Waermeaustausch PCM - Umgebung ==
  note: PQ_PCM_Umgebung = UA_PCM_Umgebung * (T_PCM - T_Umgebung_Offset)
      |
      | mit UA_PCM_Umgebung = f (v_Fahrzeug)
      | mit T_PCM_Offset = T_Umgebung + T_PCM_Offset
      |
      | -> Da die Umgebungstemperatur konstant ist, wird über T_PCM_Offset die Umgebungstemperatur um das Batteriepack manuell erhöht
  T_PCM [K] : Inport
  T_Umgebung_Offset [K] : Inport  Port=2
  v_Fahrzeug [m*s^-1] : Inport  Port=3
  1-D Lookup Table : Lookup_n-D  NumberOfTableDimensions=1  BreakpointsForDimension1=UA_PCM_Umgebung_Break_v_Fahrzeug{1}  BeginIndexSearchUsingPreviousIndexResult=on  Table=UA_PCM_Umgebung_Table{1}  ExtrapMethod=Clip  UseLastTableValue=on  InternalRulePriority=Speed  RndMeth=Simplest  InputSameDT=on
  Product1 : Product
  Subtract : Sum  Inputs=+-
  PQ_PCM_Umgebung [W] : Outport
  wires:
  v_Fahrzeug [m*s^-1]/1 -> 1-D Lookup Table/1
  Subtract/1 -> Product1/2
  1-D Lookup Table/1 -> Product1/1  "UA_PCM_Umgebung [W*K^-1]"
  Product1/1 -> PQ_PCM_Umgebung [W]/1
  T_Umgebung_Offset [K]/1 -> Subtract/2
  T_PCM [K]/1 -> Subtract/1

== system mod_sim_VTMS/Thermomanagementsystem/Batteriepack/Batteriepack(1) elektrisch/Batteriepackgrößen/Enabled Subsystem ==
  P_Verlust_Zelle_irreversibel [W] : Inport
  P_Zelle [W] : Inport  Port=2
  Enable : EnablePort
  Add1 : Sum
  Divide : Product  Inputs=/*
  Divide1 : Product  Inputs=*/
  Gain : Gain  Gain=100
  Switch : Switch  Criteria=u2 > Threshold
  eta_Batteriepack [%] : Outport
  wires:
  Gain/1 -> eta_Batteriepack [%]/1
  P_Verlust_Zelle_irreversibel [W]/1 -> Add1/1
  Add1/1 -> Divide1/1, Divide/1
  Switch/1 -> Gain/1
  Divide/1 -> Switch/1
  P_Zelle [W]/1 -> Add1/2, Divide1/2, Divide/2, Switch/2
  Divide1/1 -> Switch/3

== system mod_sim_VTMS/Thermomanagementsystem/Batteriepack/Batteriepack(1) elektrisch/Zellmodell (abgeleitet aus Batteriepackmodell -> siehe FTM)/Ohmscher Spannungsanteil und Klemmenspannung der Zelle ==
  note: Klemmenspannung der Zelle:
      |
      | U_Zelle = U_Potential + U_Ohm
      | 	      = U_Potential + R_i * I_Zelle
  I_Zelle [A] : Inport
  U_Potential [V] : Inport  Port=2
  BatPara : Inport  Port=3
  Add : Sum
  Bus Selector1 : BusSelector  OutputSignals=R_i
  Product : Product
  U_Zelle [V] : Outport
  U_Ohm [V] : Outport  Port=2
  wires:
  Bus Selector1/1 -> Product/1  "<R_i>"
  U_Potential [V]/1 -> Add/1
  BatPara/1 -> Bus Selector1/1
  Product/1 -> U_Ohm [V]/1, Add/2
  I_Zelle [A]/1 -> Product/2
  Add/1 -> U_Zelle [V]/1

== system mod_sim_VTMS/Thermomanagementsystem/Batteriepack/Batteriepack(1) elektrisch/Zellmodell (abgeleitet aus Batteriepackmodell -> siehe FTM)/Potential der Zelle ==
  note: Potential der Zelle:
      | -> Elektrischer Ersatzschaltkreis einer Zelle vereinfacht sich zum Potential der Zelle und dem ohmschen Innenwiderstand der Zelle
      |
      | U_Potential = U_SOC + U_Hysterese + U_RC1 + U_RC2
  I_Zelle [A] : Inport
  T_Zelle [°C] : Inport  Port=2
  dt [s] : Inport  Port=3
  BatState_in : Inport  Port=4
  Add : Sum  Inputs=++++
  Bus Creator : BusCreator  Inputs=5
  ECM-Parameter Look-Ups : Subsystem
  Hysteresespannung : Subsystem
  Ladezustandsabhängige Spannung : Subsystem
  SOC-Bestimmung : Subsystem
  Spannung am ersten RC-Glied : Subsystem
  Spannung am zweiten RC-Glied : Subsystem
  Terminator : Terminator
  U_Potential [V] : Outport
  BatPara : Outport  Port=2
  BatState_out : Outport  Port=3
  wires:
  dt [s]/1 -> SOC-Bestimmung/3(dt [s]), Spannung am zweiten RC-Glied/3(dt [s]), Spannung am ersten RC-Glied/3(dt [s]), Hysteresespannung/2(dt [s])
  Hysteresespannung/1(U_Hysterese [V]) -> Add/2, Bus Creator/3  "U_Hysterese"
  I_Zelle [A]/1 -> ECM-Parameter Look-Ups/2(I_Zelle [A]), SOC-Bestimmung/4(I_Zelle [A]), Spannung am zweiten RC-Glied/4(I_Zelle [A]), Spannung am ersten RC-Glied/4(I_Zelle [A]), Hysteresespannung/3(I_Zelle [A])
  Spannung am ersten RC-Glied/1(U_RC1 [V]) -> Add/3, Bus Creator/4  "U_RC1"
  ECM-Parameter Look-Ups/2(BatPara_Pulses) -> BatPara/1, Spannung am zweiten RC-Glied/2(BatPara), Spannung am ersten RC-Glied/2(BatPara), Ladezustandsabhängige Spannung/2(BatPara), SOC-Bestimmung/2(BatPara)
  Spannung am zweiten RC-Glied/1(U_RC2 [V]) -> Add/4, Bus Creator/5  "U_RC2"
  Ladezustandsabhängige Spannung/1(U_SOC [V]) -> Add/1, Bus Creator/2  "U_SOC"
  Bus Creator/1 -> BatState_out/1
  SOC-Bestimmung/1(SOC [-]) -> Bus Creator/1, Ladezustandsabhängige Spannung/1(SOC [-])  "SOC"
  T_Zelle [°C]/1 -> ECM-Parameter Look-Ups/1(T_Zelle [°C])
  BatState_in/1 -> ECM-Parameter Look-Ups/3(BatState), Spannung am zweiten RC-Glied/1(BatState_In), Spannung am ersten RC-Glied/1(BatState_In), Hysteresespannung/1(BatState_In), SOC-Bestimmung/1(BatState_In)
  ECM-Parameter Look-Ups/1(BatPara_EIS) -> Terminator/1
  Add/1 -> U_Potential [V]/1

== system mod_sim_VTMS/Thermomanagementsystem/Batteriepack/Batteriepack(1) elektrisch/Zellmodell (abgeleitet aus Batteriepackmodell -> siehe FTM)/Verlustleistung der Zelle ==
  note: Verlustleistung der Zelle:
      |
      | P_Verlust_Zelle = P_Verlust_Zelle_irreversibel + P_Verlust_Zelle_reversibel
  T_Zelle [°C] : Inport
  I_Zelle [A] : Inport  Port=2
  U_Ohm [V] : Inport  Port=3
  BatPara : Inport  Port=4
  BatState : Inport  Port=5
  Bus Selector : BusSelector  OutputSignals=U_RC1,U_RC2
  "Irreversible Verlustleistung " : Subsystem
  Reversible Verlustleistung : Subsystem
  P_Verlust_Zelle_irreversibel [W] : Outport
  P_Verlust_Zelle_reversibel [W] : Outport  Port=2
  wires:
  BatPara/1 -> Reversible Verlustleistung/2(BatPara)
  I_Zelle [A]/1 -> "Irreversible Verlustleistung "/4(I_Zelle [A]), Reversible Verlustleistung/1(I_Zelle [A])
  BatState/1 -> Bus Selector/1
  Bus Selector/1 -> "Irreversible Verlustleistung "/2(U_RC1 [V])  "<U_RC1>"
  Bus Selector/2 -> "Irreversible Verlustleistung "/3(U_RC2 [V])  "<U_RC2>"
  U_Ohm [V]/1 -> "Irreversible Verlustleistung "/1(U_Ohm [V])
  Reversible Verlustleistung/1(P_Verlust_Zelle_reversibel  [W]) -> P_Verlust_Zelle_reversibel [W]/1
  T_Zelle [°C]/1 -> Reversible Verlustleistung/3(T_Zelle [°C])
  "Irreversible Verlustleistung "/1(P_Verlust_Zelle_irreversibel [W]) -> P_Verlust_Zelle_irreversibel [W]/1

== system mod_sim_VTMS/Thermomanagementsystem/Batteriepack/Batteriepack(1) elektrisch/Zellmodell (abgeleitet aus Batteriepackmodell -> siehe FTM)/dt ==
  note: Zu Beginn ist dt=0
      | -> Das initiale Potential ergibt sich korrekterweise aus dem initialen SOC und damit der initialen ladezustandsabhängigen Spannung, aus der initialen Hysteresespannung, aus der initialen Spannung am ersten RC-Glied und aus der initialen Spannung am zweiten RC-Glied
  Clock : Clock
  Subtract : Sum  Inputs=+-
  Unit Delay : UnitDelay  SampleTime=-1
  dt [s] : Outport
  wires:
  Unit Delay/1 -> Subtract/2
  Clock/1 -> Unit Delay/1, Subtract/1
  Subtract/1 -> dt [s]/1

== system mod_sim_VTMS/Thermomanagementsystem/Fluid/Bestimmung PV_Kuehlkreislauf/Kuehlkreislauf/Steuerung Pumpe ==
  note: Steuerung Pumpe:
      | -> Eine Pumpe wird über den Volumenstrom im Kühlkreislauf gesteuert
      | -> Die Steuerung des Volumenstroms in einem Kühlkreislauf erfolgt über die maximale Temperatur der zu temperierenden Komponenten in dem entsprechenden Kühlkreislauf
      | -> Abhängig von der maximalen Temperatur der zu temperierenden Komponenten in dem entsprechenden Kühlkreislauf stellt sich ein bestimmter Volumenstrom im Kühlkreislauf ein
      | -> Die zu temperierenden Komponenten in einem Kühlkreislauf können die E-Maschine, die Leistungselektronik und das Batteriepack sein
      | -> Bei der Leistungselektronik dient die Temperatur der Gehäuse der MOSFET als Referenz
      |
      | PV_Kuehlkreislauf = f (T_Komponente_max)
      |
      | -> Bei einer realen Steuerung existiert eine Totzeit
      | -> Totzeit = Zeitspanne zwischen der Signaländerung am Systemeingang und der Signalantwort am Systemausgang
      | -> Die Totzeit der Steuerung der Pumpen wird vom Anwender in MATLAB festgelegt und ist hier über den Block "Delay" realisiert
      | -> Da das Thermomanagementsystemmodell zeitdiskret ausgewertet wird, kann es sein, dass die Totzeit der Steuerung der Pumpen nicht exakt eingehalten wird
      | -> Dies tritt für den Fall ein, wenn die Totzeit der Steuerung der Pumpen kein Vielfaches vom Zeitschritt der Simulation ist
      | -> Für diesen Fall stellt sich die Signalantwort am Systemausgang zum darauffolgenden Auswertungszeitpunkt ein
      |
      | -> Wenn in einem Kühlkreislauf keine zu temperierende Komponente konfiguriert ist, existiert keine maximale Temperatur der zu temperierenden Komponenten in dem entsprechenden Kühlkreislauf
      | -> Diese Größe ist dann während der Simulation durchgehend = 0K
      | -> Deswegen wird für den Volumenstrom in dem entsprechenden Kühlkreislauf während der Simulation durchgehend der untere Grenzwert des vorgegebenen Kennfelds herangezogen
  EMaschine_Output : Inport
  Leistungselektronik_Output : Inport  Port=2
  Batteriepack_Output : Inport  Port=3
  Bus Selector : BusSelector  OutputSignals=T_EMaschine_Getriebe [K].T_EMaschine [K]
  Bus Selector1 : BusSelector  OutputSignals=T_Leistungselektronik [K].T_c [K]
  Bus Selector2 : BusSelector  OutputSignals=T_Batteriepack [K]
  Delay : Delay  DelayLength=ceil(Totzeit_Steuerung_Pumpe/delta_t)  InitialConditionSource=Input port  InitialCondition=0
      settings: InputPortMap=u0,p4
  From Workspace : FromWorkspace  VariableName=[0,0]  SampleTime=0
  Max : MinMax  Function=max
  n-D Lookup Table : Lookup_n-D  NumberOfTableDimensions=1  BreakpointsForDimension1=0  BreakpointsForDimension3=[5, 7]  Table=0  ExtrapMethod=Clip  UseLastTableValue=on  InternalRulePriority=Speed  RndMeth=Simplest  InputSameDT=on
  PV_Kuehlkreislauf [m^3*s^-1] : Outport
  wires:
  n-D Lookup Table/1 -> Delay/2, Delay/1
  Leistungselektronik_Output/1 -> Bus Selector1/1
  EMaschine_Output/1 -> Bus Selector/1
  Batteriepack_Output/1 -> Bus Selector2/1
  Max/1 -> n-D Lookup Table/1  "T_Komponente_max [K]"
  From Workspace/1 -> Max/1
  Delay/1 -> PV_Kuehlkreislauf [m^3*s^-1]/1

== system mod_sim_VTMS/Thermomanagementsystem/Fluid/Bestimmung Zustand_Ventil/Ventil/Steuerung Ventil ==
  note: Steuerung Dreiwegeventil:
      | -> Ein Dreiwegeventil wird über den Zustand des Dreiwegeventils gesteuert
      | -> Die Steuerung des Zustands des Dreiwegeventils erfolgt über die Temperatur der Kühlflüssigkeit bzgl. des Knotens des n. finiten Volumens der Fluid_Komponente, die bei der Definition des Dreiwegeventils bei Ventil_nach festgelegt ist
      | -> Abhängig von der Temperatur der Kühlflüssigkeit bzgl. des Knotens des n. finiten Volumens der Fluid_Komponente, die bei der Definition des Dreiwegeventils bei Ventil_nach festgelegt ist, stellt sich ein bestimmter Zustand des Dreiwegeventils ein
      |
      | Zustand_Ventil = f (T_FinitesVolumen_Ventil_nach_n)
      |
      | -> Bei einer realen Steuerung existiert eine Totzeit
      | -> Totzeit = Zeitspanne zwischen der Signaländerung am Systemeingang und der Signalantwort am Systemausgang
      | -> Die Totzeit der Steuerung der Dreiwegeventile wird vom Anwender in MATLAB festgelegt und ist hier über den Block "Delay" realisiert
      | -> Da das Thermomanagementsystemmodell zeitdiskret ausgewertet wird, kann es sein, dass die Totzeit der Steuerung der Dreiwegeventile nicht exakt eingehalten wird
      | -> Dies tritt für den Fall ein, wenn die Totzeit der Steuerung der Dreiwegeventile kein Vielfaches vom Zeitschritt der Simulation ist
      | -> Für diesen Fall stellt sich die Signalantwort am Systemausgang zum darauffolgenden Auswertungszeitpunkt ein
  Fluid_Schlauch_Output : Inport
  Bus Selector : BusSelector  OutputSignals=signal1
  Delay : Delay  DelayLength=ceil(Totzeit_Steuerung_Ventil/delta_t)  InitialConditionSource=Input port  InitialCondition=0
      settings: InputPortMap=u0,p4
  Selector_n : Selector  IndexOptions=Index vector (dialog)  Indices=1  OutputSizes=1
  n-D Lookup Table : Lookup_n-D  NumberOfTableDimensions=1  BreakpointsForDimension1=0  BreakpointsForDimension3=[5, 7]  Table=0  ExtrapMethod=Clip  UseLastTableValue=on  InternalRulePriority=Speed  RndMeth=Simplest  InputSameDT=on
  Zustand_Ventil [-] : Outport
  wires:
  Fluid_Schlauch_Output/1 -> Bus Selector/1
  n-D Lookup Table/1 -> Delay/2, Delay/1
  Selector_n/1 -> n-D Lookup Table/1  "T_FinitesVolumen_Ventil_nach_n [K]"
  Bus Selector/1 -> Selector_n/1  "<signal1>"
  Delay/1 -> Zustand_Ventil [-]/1

== system mod_sim_VTMS/Thermomanagementsystem/Fluid/Fluid_Komponente thermisch/Bestimmung PV_Kuehlfluessigkeit/Ventil ==
  Zustand_Ventil [-] : Inport
  Bus Selector : BusSelector  OutputSignals=signal1
  Constant : Constant  VectorParams1D=off
  Hauptpfad : Constant  Value=0  VectorParams1D=off
  Subtract : Sum  Inputs=+-
  Switch : Switch  Criteria=u2 > Threshold
  PV_Kuehlkreislauf_Faktor_Ventil [-] : Outport
  wires:
  Constant/1 -> Subtract/1
  Subtract/1 -> Switch/1
  Hauptpfad/1 -> Switch/2
  Bus Selector/1 -> Subtract/2, Switch/3  "<signal1>"
  Switch/1 -> PV_Kuehlkreislauf_Faktor_Ventil [-]/1
  Zustand_Ventil [-]/1 -> Bus Selector/1

== system mod_sim_VTMS/Thermomanagementsystem/Kühler/Kuehler thermisch/Bestimmung v_Kuehlerluefter/Steuerung Kuehlerluefter ==
  note: Steuerung Kühlerlüfter:
      | -> Ein Kühlerlüfter wird über die Luftgeschwindigkeit des Kühlerlüfters gesteuert
      | -> Die Steuerung der Luftgeschwindigkeit eines Kühlerlüfters erfolgt über die Temperatur der Kühlflüssigkeit bzgl. des Knotens des 1. oder n. finiten Volumens des Strömungsgebiets des entsprechenden Kühlers
      | -> Abhängig von der Temperatur der Kühlflüssigkeit bzgl. des Knotens des 1. oder n. finiten Volumens des Strömungsgebiets des entsprechenden Kühlers stellt sich eine bestimmte Luftgeschwindigkeit des Kühlerlüfters ein
      | -> Über den Block "Manual Switch" kann manuell zwischen der Temperatur der Kühlflüssigkeit bzgl. des Knotens des 1. (Block "Selector_1") und des n. (Block "Selector_n") finiten Volumens des Strömungsgebiets des entsprechenden Kühlers umgeschaltet werden
      |
      | v_Kuehlerluefter = f (T_FinitesVolumen_Kuehler_1) oder f (T_FinitesVolumen_Kuehler_n)
      |
      | -> Bei einer realen Steuerung existiert eine Totzeit
      | -> Totzeit = Zeitspanne zwischen der Signaländerung am Systemeingang und der Signalantwort am Systemausgang
      | -> Die Totzeit der Steuerung der Kühlerlüfter wird vom Anwender in MATLAB festgelegt und ist hier über den Block "Delay" realisiert
      | -> Da das Thermomanagementsystemmodell zeitdiskret ausgewertet wird, kann es sein, dass die Totzeit der Steuerung der Kühlerlüfter nicht exakt eingehalten wird
      | -> Dies tritt für den Fall ein, wenn die Totzeit der Steuerung der Kühlerlüfter kein Vielfaches vom Zeitschritt der Simulation ist
      | -> Für diesen Fall stellt sich die Signalantwort am Systemausgang zum darauffolgenden Auswertungszeitpunkt ein
  T_FinitesVolumen [K] : Inport
  Delay : Delay  DelayLength=ceil(Totzeit_Steuerung_Kuehlerluefter/delta_t)  InitialConditionSource=Input port  InitialCondition=0
      settings: InputPortMap=u0,p4
  Manual Switch : ManualSwitch
  Selector_1 : Selector  IndexOptions=Index vector (dialog)  Indices=1  OutputSizes=1
  Selector_n : Selector  IndexOptions=Index vector (dialog)  Indices=1  OutputSizes=1
  n-D Lookup Table : Lookup_n-D  NumberOfTableDimensions=1  BreakpointsForDimension1=0  BreakpointsForDimension3=[5, 7]  Table=0  ExtrapMethod=Clip  UseLastTableValue=on  InternalRulePriority=Speed  RndMeth=Simplest  InputSameDT=on
  v_Kuehlerluefter [m*s^-1] : Outport
  wires:
  T_FinitesVolumen [K]/1 -> Selector_n/1, Selector_1/1
  n-D Lookup Table/1 -> Delay/1, Delay/2
  Manual Switch/1 -> n-D Lookup Table/1
  Selector_n/1 -> Manual Switch/2  "T_FinitesVolumen_Kuehler_n [K]"
  Selector_1/1 -> Manual Switch/1  "T_FinitesVolumen_Kuehler_1 [K]"
  Delay/1 -> v_Kuehlerluefter [m*s^-1]/1
